simulink model "Accelerator"  (R2022b)
settings: Solver=VariableStepAuto  StartTime=0.0  StopTime=20  RelTol=1e-3
libraries: simulink x5, slpidlib x1
settings Model: Creator=david  LastModifiedBy=david
settings SolverCC: ZeroCrossAlgorithm=Adaptive
settings DebuggingCC: IgnoredZcDiagnostic=none  UnconnectedInputMsg=warning  UnconnectedOutputMsg=warning  UnconnectedLineMsg=warning
settings ModelReferenceCC: EnableRefExpFcnMdlSchedulingChecks=on
settings RTWCC: DLArmComputeVersion=19.05

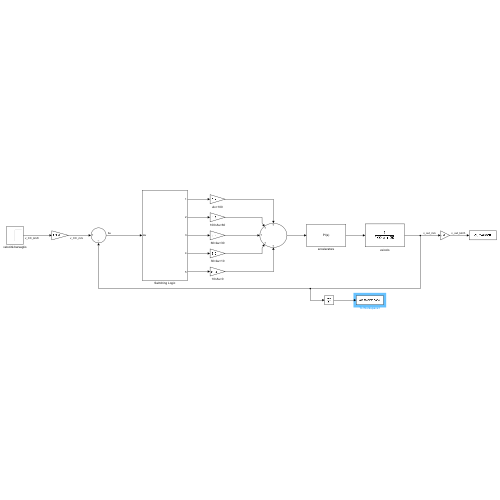
[thumbnail: Simulink's stored preview of the top-level diagram]
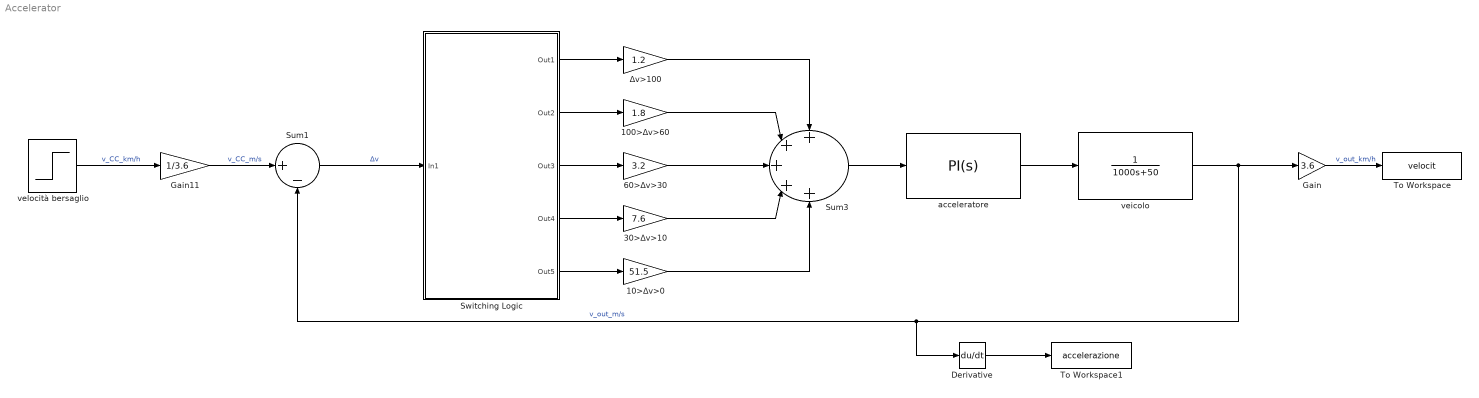
== system Accelerator ==
  100>Δv>60 : Gain  Gain=1.8
  10>Δv>0 : Gain  Gain=51.5
  30>Δv>10 : Gain  Gain=7.6
  60>Δv>30 : Gain  Gain=3.2
  Derivative : Derivative
  Gain : Gain  Gain=3.6
  Gain11 : Gain  Gain=1/3.6
  Sum1 : Sum  Inputs=|+-
  Sum3 : Sum  Inputs=+++++
  Switching Logic : Subsystem
  To Workspace : ToWorkspace  VariableName=velocit  SampleTime=-1
  To Workspace1 : ToWorkspace  VariableName=accelerazione  SampleTime=-1
  acceleratore : slpidlib/PID Controller  Controller=PI  Form=Parallel  TimeDomain=Continuous-time  UseExternalTs=off  SampleTime=-1  IntegratorMethod=Forward Euler  FilterMethod=Forward Euler  ControllerParametersSource=internal  P=20  I=1  UseKiTs=off  D=0  N=100  UseFilter=on  TunerSelectOption=Transfer Function Based (PID Tuner App)  InitialConditionSource=internal  InitialConditionForIntegrator=0  InitialConditionForFilter=0  DifferentiatorICPrevScaledInput=0  ExternalReset=none  TrackingMode=off  Kt=1  LimitOutput=off  SatLimitsSource=internal  UpperSaturationLimit=inf  LowerSaturationLimit=-inf  LinearizeAsGain=on  AntiWindupMode=none  Kb=1  LimitIntegrator=off  UpperIntegratorSaturationLimit=inf  LowerIntegratorSaturationLimit=-inf  POutMin=[]  POutMax=[]  IOutMin=[]  IOutMax=[]  DOutMin=[]  DOutMax=[]  NOutMin=[]  NOutMax=[]  SumOutMin=[]  SumOutMax=[]  SaturationOutMin=[]  SaturationOutMax=[]  PParamMin=[]  PParamMax=[]  IParamMin=[]  IParamMax=[]  DParamMin=[]  DParamMax=[]  NParamMin=[]  NParamMax=[]  KbParamMin=[]  KbParamMax=[]  KtParamMin=[]  KtParamMax=[]  KbOutMin=[]  KbOutMax=[]  KtOutMin=[]  KtOutMax=[]  IntegratorOutMin=[]  IntegratorOutMax=[]  FilterOutMin=[]  FilterOutMax=[]  SumI1OutMin=[]  SumI1OutMax=[]  SumI2OutMin=[]  SumI2OutMax=[]  SumI3OutMin=[]  SumI3OutMax=[]  SumI4OutMin=[]  SumI4OutMax=[]  SumDOutMin=[]  SumDOutMax=[]  DifferentiatorOutMin=[]  DifferentiatorOutMax=[]  FilterDiffOutCoefMin=[]  FilterDiffOutCoefMax=[]  ReciprocalOutMin=[]  ReciprocalOutMax=[]  SumDenOutMin=[]  SumDenOutMax=[]  SumNumOutMin=[]  SumNumOutMax=[]  DivideOutMin=[]  DivideOutMax=[]  UdiffTsProdOutMin=[]  UdiffTsProdOutMax=[]  NTsProdOutMin=[]  NTsProdOutMax=[]  UintegralTsProdOutMin=[]  UintegralTsProdOutMax=[]  UngainTsProdOutMin=[]  UngainTsProdOutMax=[]  ClampingZeroOutDataTypeStr=Inherit: Inherit via back propagation  ClampingZeroOutMin=[]  ClampingZeroOutMax=[]  FilterDenConstantOutDataTypeStr=Inherit: Inherit via back propagation  FilterDenConstantOutMin=[]  FilterDenConstantOutMax=[]  PCopyOutDataTypeStr=Inherit: Inherit via back propagation  PCopyOutMin=[]  PCopyOutMax=[]  NCopyOutDataTypeStr=Inherit: Inherit via back propagation  NCopyOutMin=[]  NCopyOutMax=[]  IntegratorContinuousStateAttributes=''  IntegratorStateMustResolveToSignalObject=off  IntegratorRTWStateStorageClass=Auto  FilterContinuousStateAttributes=''  FilterStateMustResolveToSignalObject=off  FilterRTWStateStorageClass=Auto  ParallelPVariant=InternalParameters  IdealPVariant=Disabled  IVariant=InternalParameters  DVariant=Disabled  IntegratorVariant=Continuous  SatVariant=Disabled  AWVariant=Passthrough  PCopyVariant=Disabled  TRVariant=Disabled  FdbkBlocksVariant=Forward  IdealPFdbkVariant=Disabled  SatFdbkVariant=Disabled  DerivativeFilterVariant=Disabled  NVariant=Disabled  NCopyVariant=Disabled_SignalSpec  FilterICVariant=Disabled  IntegratorICVariant=InternalICs  ExternalResetVariant=Disabled  TRSumVariant=Passthrough  SumFdbkVariant=Disabled  SumVariant=Sum_PI  TsampFilterVariant=InternalTs  TsampNgainVariant=Passthrough  TsampIntegralVariant=Passthrough  ExternalSaturationOutDataTypeStr=Inherit: Same as second input
  veicolo : TransferFcn  Denominator=[1000 50]
  velocità bersaglio : Step  Time=0  After=15  SampleTime=0.0001
  Δv>100 : Gain  Gain=1.2
  wires:
  Gain/1 -> To Workspace/1  "v_out_km/h"
  Sum1/1 -> Switching Logic/1(In1)  "Δv"
  veicolo/1 -> Gain/1, Derivative/1, Sum1/2  "v_out_m/s"
  Sum3/1 -> acceleratore/1
  10>Δv>0/1 -> Sum3/5
  30>Δv>10/1 -> Sum3/4
  100>Δv>60/1 -> Sum3/2
  Δv>100/1 -> Sum3/1
  Gain11/1 -> Sum1/1  "v_CC_m/s"
  velocità bersaglio/1 -> Gain11/1  "v_CC_km/h"
  acceleratore/1 -> veicolo/1
  Derivative/1 -> To Workspace1/1
  60>Δv>30/1 -> Sum3/3
  Switching Logic/1(Out1) -> Δv>100/1
  Switching Logic/2(Out2) -> 100>Δv>60/1
  Switching Logic/3(Out3) -> 60>Δv>30/1
  Switching Logic/4(Out4) -> 30>Δv>10/1
  Switching Logic/5(Out5) -> 10>Δv>0/1

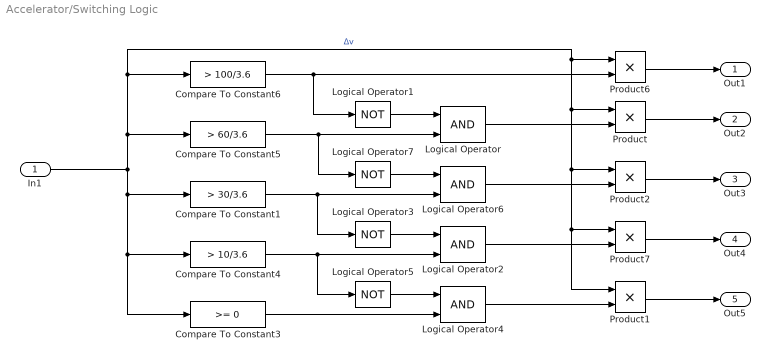
== system Accelerator/Switching Logic ==
  In1 : Inport
  Compare To Constant1 : simulink/Logic and Bit Operations/Compare To Constant  relop=>  const=30/3.6  OutDataTypeStr=boolean
  Compare To Constant3 : simulink/Logic and Bit Operations/Compare To Constant  relop=>=  const=0  OutDataTypeStr=boolean
  Compare To Constant4 : simulink/Logic and Bit Operations/Compare To Constant  relop=>  const=10/3.6  OutDataTypeStr=boolean
  Compare To Constant5 : simulink/Logic and Bit Operations/Compare To Constant  relop=>  const=60/3.6  OutDataTypeStr=boolean
  Compare To Constant6 : simulink/Logic and Bit Operations/Compare To Constant  relop=>  const=100/3.6  OutDataTypeStr=boolean
  Logical Operator{,2,4,6} (4 alike) : Logic  AllPortsSameDT=off  OutDataTypeStr=boolean
  Logical Operator{1,3,5,7} (4 alike) : Logic  Operator=NOT  AllPortsSameDT=off  OutDataTypeStr=boolean
  Product{,1..2,6..7} (5 alike) : Product
  Out1 : Outport
  Out2 : Outport  Port=2
  Out3 : Outport  Port=3
  Out4 : Outport  Port=4
  Out5 : Outport  Port=5
  wires:
  Compare To Constant1/1 -> Logical Operator3/1, Logical Operator6/2
  Logical Operator6/1 -> Product2/2
  Compare To Constant3/1 -> Logical Operator4/2
  Logical Operator1/1 -> Logical Operator/1
  Product2/1 -> Out3/1
  Product6/1 -> Out1/1
  Logical Operator/1 -> Product/2
  Compare To Constant5/1 -> Logical Operator7/1, Logical Operator/2
  Product1/1 -> Out5/1
  Logical Operator7/1 -> Logical Operator6/1
  Logical Operator2/1 -> Product7/2
  Compare To Constant4/1 -> Logical Operator5/1, Logical Operator2/2
  Logical Operator4/1 -> Product1/2
  Logical Operator3/1 -> Logical Operator2/1
  Logical Operator5/1 -> Logical Operator4/1
  Compare To Constant6/1 -> Product6/2, Logical Operator1/1
  In1/1 -> Compare To Constant5/1, Product/1, Product2/1, Product7/1, Product1/1, Product6/1, Compare To Constant6/1, Compare To Constant1/1, Compare To Constant3/1, Compare To Constant4/1  "Δv"
  Product/1 -> Out2/1
  Product7/1 -> Out4/1
